simulink model "Simulink_model"  (R2018a)
settings: Solver=VariableStepAuto  StartTime=0.0  StopTime=10.0  RelTol=1e-3  EnableMultiTasking=on
libraries: commanapbnd3 x2, phasedtxrxlib x2, commchan3 x1, commrflib2 x1, dspvision x1
settings Model: Creator=hazi  LastModifiedBy=ASUS
settings OptimizationCC: LifeSpan=inf
settings DebuggingCC: SFUnexpectedBacktrackingDiag=warning  SFNoUnconditionalDefaultTransitionDiag=warning  SFExecutionAtInitializationDiag=none
settings CodeAppCC: StateflowObjectComments=on
settings GRTTargetCC: TargetLangStandard=C89/C90 (ANSI)  GeneratePreprocessorConditionals=Disable all
settings ConfigComp: CovMetricSettings=dw  CovHtmlReporting=on  CovSaveCumulativeToWorkspaceVar=on  CovSaveSingleToWorkspaceVar=on  CovExternalEMLEnable=off

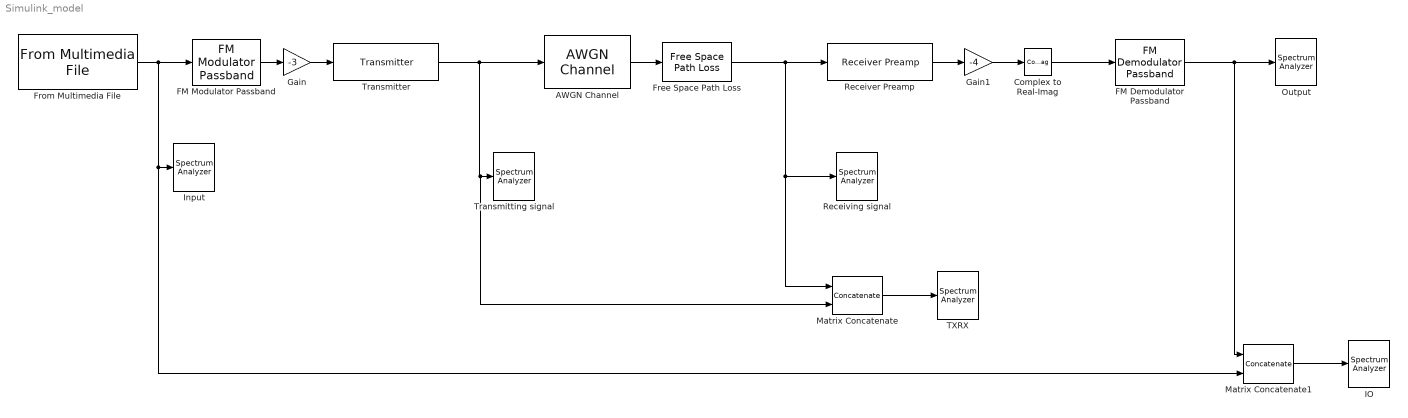
== system Simulink_model ==
  AWGN Channel : commchan3/AWGN Channel  InputProcessing=Columns as channels (frame based)  seed=67  noiseMode="Signal to noise ratio  (Eb/No)"  EbNodB=10  EsNodB=10  SNRdB=10  bitsPerSym=1  Ps=1  Tsym=1  variance=1
  Complex to Real-Imag : ComplexToRealImag  Output=Real
  FM Demodulator Passband : commanapbnd3/FM Demodulator Passband  Fc=50000000000  Ph=0  Kc=3999  Ho=100
      settings: SourceProductName=Communications System Toolbox  SourceProductBaseCode=CM
  FM Modulator Passband : commanapbnd3/FM Modulator Passband  Fc=50000000000  Ph=0  Kc=3999
      settings: SourceProductName=Communications System Toolbox  SourceProductBaseCode=CM
  Free Space Path Loss : commrflib2/Free Space Path Loss  mode=Decibels  dB=207.6  d=0.100  fc=1920
      settings: SourceProductName=Communications System Toolbox  SourceProductBaseCode=CM
  From Multimedia File : dspvision/From Multimedia File  inputFilename=C:\Users\ASUS\Desktop\Telecom Assignment\sound.wav  loop=on  numPlays=1  outputStreams=Audio only  videoDataType=single  audioDataType=double  inheritSampleTime=on  userDefinedSampleTime=1/30  noAudioOutput=off  isIntensityVideo=off  fourcc=RGB  colorVideoFormat=Separate color signals  outputEOF=off  dataOrg=Column-major  audioFrameSize=1  computeAudioFrameSize=off  outSamplingMode=Sample based
      settings: SourceProductBaseCode=VP
  Gain : Gain  Gain=-3
  Gain1 : Gain  Gain=-4
  IO : SpectrumAnalyzer
  "Input " : SpectrumAnalyzer
  Matrix Concatenate : Concatenate  Mode=Multidimensional array  ConcatenateDimension=2
  Matrix Concatenate1 : Concatenate  Mode=Multidimensional array  ConcatenateDimension=2
  "Output " : SpectrumAnalyzer
  Receiver Preamp : phasedtxrxlib/Receiver Preamp  Gain=54.77  LossFactor=0  NoiseMethod=Noise power  NoiseFigure=0  ReferenceTemperature=290  SampleRateFromInputCheckbox=on  SampleRate=1e6  NoisePower=0  EnableInputPort=off  PhaseNoiseInputPort=off  SeedSource=Property  Seed=randi(65535,1)  SimulateUsing=Interpreted execution
      settings: SourceProductName=Phased Array System Toolbox  SourceProductBaseCode=AR
  Receiving signal : SpectrumAnalyzer
  "TXRX " : SpectrumAnalyzer
  Transmitter : phasedtxrxlib/Transmitter  PeakPower=5000  Gain=30  LossFactor=0  InUseOutputPort=off  CoherentOnTransmit=on  PhaseNoiseOutputPort=off  SeedSource=Property  Seed=randi(65535,1)  SimulateUsing=Interpreted execution
      settings: SourceProductName=Phased Array System Toolbox  SourceProductBaseCode=AR
  Transmitting signal : SpectrumAnalyzer
  wires:
  FM Modulator Passband/1 -> Gain/1
  Gain/1 -> Transmitter/1
  Transmitter/1 -> Matrix Concatenate/2, Transmitting signal/1, AWGN Channel/1
  AWGN Channel/1 -> Free Space Path Loss/1
  Receiver Preamp/1 -> Gain1/1
  Free Space Path Loss/1 -> Receiver Preamp/1, Matrix Concatenate/1, Receiving signal/1
  Gain1/1 -> Complex to Real-Imag/1
  Complex to Real-Imag/1 -> FM Demodulator Passband/1
  Matrix Concatenate/1 -> "TXRX "/1
  FM Demodulator Passband/1 -> Matrix Concatenate1/1, "Output "/1
  Matrix Concatenate1/1 -> IO/1
  From Multimedia File/1 -> Matrix Concatenate1/2, "Input "/1, FM Modulator Passband/1
